simulink model "radial_magnetic_bearing_revised"  (R2021a)
settings: Solver=VariableStepAuto  StartTime=0.0  StopTime=10  RelTol=1e-3
values from neighbouring files (symbols this model uses):
  Ar = [zeros(4) eye(4); zeros(4) -G/M]    [radial_amb.m]
  Br = [zeros(4);B/M]    [radial_amb.m]
  Cr = [C zeros(4)]    [radial_amb.m]
  Dr = zeros(4)    [radial_amb.m]
  Ki = eye(4)*ki    [radial_amb.m]
  KLQR = Nbar    [radial_amb.m]
  Kss = (B*Ks*B')'    [radial_amb.m]
  P0ramb = diag(100*ones(1,8))    [radial_amb.m]
  Qramb = diag(10^-14*ones(1,8))    [radial_amb.m]
  Rramb = diag(10^-14*ones(1,4))    [radial_amb.m]
  sys_dr = c2d(Hsi,dT,'zoh')    [radial_amb.m]
  Tr = inv(T)    [radial_amb.m]
  x0ramb = [0;0;0;0;0;0;0;0]    [radial_amb.m]
libraries: simulink x32
settings Model: Creator=macbookpro  LastModifiedBy=macbookpro

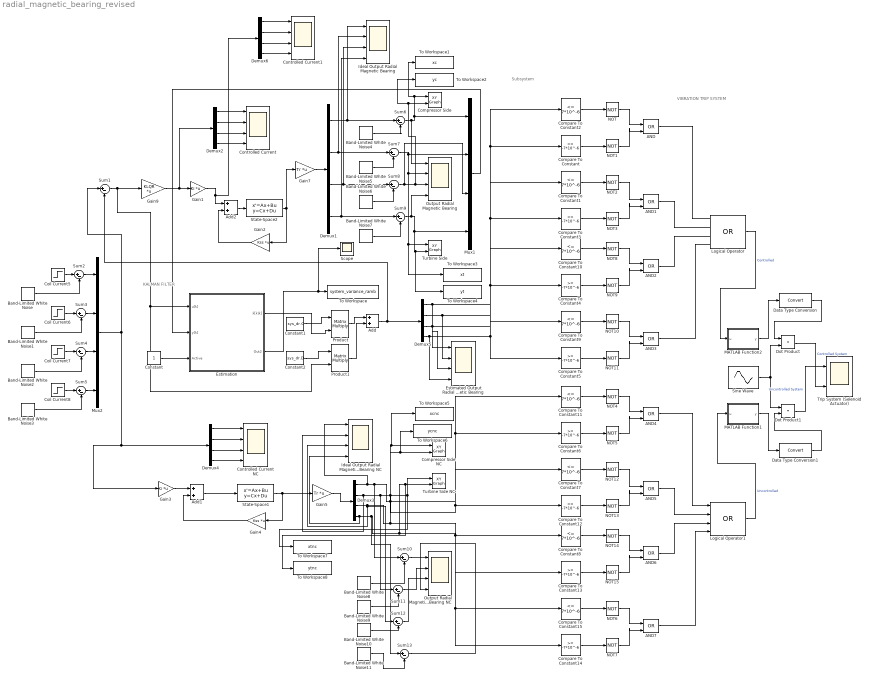
== system radial_magnetic_bearing_revised ==
  note: Subsystem
  note: KALMAN FILTER
  note: VIBRATION TRIP SYSTEM
  AND{,1..7} (8 alike) : Logic  Operator=OR  IconShape=distinctive  AllPortsSameDT=off  OutDataTypeStr=boolean
  Add : Sum
  Add1 : Sum
  Add2 : Sum
  Band-Limited White Noise{,1..3} (4 alike) : simulink/Sources/Band-Limited White Noise  Cov=[0.01]  Ts=0.1  seed=[23341]
  Band-Limited White Noise{4..11} (8 alike) : simulink/Sources/Band-Limited White Noise  Cov=[10^-14]  Ts=0.1  seed=[23341]
  Coil Current{5..8} (4 alike) : Step  After=0.5  SampleTime=0
  Compare To Constant{,3..6,12..14} (8 alike) : simulink/Logic and Bit Operations/Compare To Constant  relop=>=  const=-7*10^-6  OutDataTypeStr=boolean
  Compare To Constant{1..2,7..11,15} (8 alike) : simulink/Logic and Bit Operations/Compare To Constant  relop=<=  const=7*10^-6  OutDataTypeStr=boolean
  "Compressor Side " : simulink/Sinks/XY Graph  xmin=10*-10^-6  xmax=10*10^-6  ymin=10*-10^-6  ymax=10*10^-6  st=0.1
  Compressor Side NC : simulink/Sinks/XY Graph  xmin=10*-10^-6  xmax=10*10^-6  ymin=10*-10^-6  ymax=10*10^-6  st=0.1
  Constant : Constant
  Constant1 : Constant  Value=sys_dr.C  VectorParams1D=off
  Constant2 : Constant  Value=sys_dr.D  VectorParams1D=off
  Controlled Current : Scope  NumInputPorts=4
  Controlled Current NC : Scope  NumInputPorts=4
  Controlled Current1 : Scope  NumInputPorts=4
  Data Type Conversion : DataTypeConversion
  Data Type Conversion1 : DataTypeConversion
  Demux{1..6} (6 alike) : Demux
  Dot Product : DotProduct  InputSameDT=on  OutDataTypeStr=Inherit: Inherit via internal rule
  Dot Product1 : DotProduct  InputSameDT=on  OutDataTypeStr=Inherit: Inherit via internal rule
  Estimated Output Radial Magnetic Bearing : Scope  NumInputPorts=4
  Estimation : Subsystem
  Gain1 : Gain  Gain=Ki  Multiplication=Matrix(K*u)
  Gain2 : Gain  Gain=Kss  Multiplication=Matrix(K*u)
  Gain3 : Gain  Gain=Ki  Multiplication=Matrix(K*u)
  Gain4 : Gain  Gain=Kss  Multiplication=Matrix(K*u)
  Gain5 : Gain  Gain=Tr  Multiplication=Matrix(K*u)
  Gain7 : Gain  Gain=Tr  Multiplication=Matrix(K*u)
  Gain9 : Gain  Gain=KLQR  Multiplication=Matrix(K*u)
  Ideal Output Radial Magnetic Bearing : Scope  NumInputPorts=4
  Ideal Output Radial Magnetic Bearing NC : Scope  NumInputPorts=4
  Logical Operator : Logic  Operator=OR  Inputs=4  IconShape=distinctive  AllPortsSameDT=off  OutDataTypeStr=boolean
  Logical Operator1 : Logic  Operator=OR  Inputs=4  IconShape=distinctive  AllPortsSameDT=off  OutDataTypeStr=boolean
  MATLAB Function1 : MATLAB Function  TreatAsAtomicUnit=on
  MATLAB Function2 : MATLAB Function  TreatAsAtomicUnit=on
  Mux1 : Mux
  Mux2 : Mux
  NOT{,1..15} (16 alike) : Logic  Operator=NOT  IconShape=distinctive  AllPortsSameDT=off  OutDataTypeStr=boolean
  Output Radial Magnetic Bearing : Scope  NumInputPorts=4
  Output Radial Magnetic Bearing NC : Scope  NumInputPorts=4
  Product : Product  Multiplication=Matrix(*)
  Product1 : Product  Multiplication=Matrix(*)
  Scope : Scope
  Sine Wave : Sin  Amplitude=220  Frequency=60  SampleTime=0
  State-Space1 : StateSpace  A=Ar  B=Br  C=Cr  D=Dr  InitialCondition=0
  State-Space2 : StateSpace  A=Ar  B=Br  C=Cr  D=Dr  InitialCondition=10^-7*[1.5 1.5 1.5 1.5 1.5 1.5 1.5 1.5]  ContinuousStateAttributes='posisition'
  Sum{1..13} (13 alike) : Sum  Inputs=|+-
  To Workspace : ToWorkspace  VariableName=system_variance_ramb  SampleTime=-1
      settings: MaxDataPoints=1
  To Workspace1 : ToWorkspace  VariableName=xc  SaveFormat=Timeseries  SampleTime=-1
  To Workspace2 : ToWorkspace  VariableName=yc  SaveFormat=Timeseries  SampleTime=-1
  To Workspace3 : ToWorkspace  VariableName=xt  SaveFormat=Timeseries  SampleTime=-1
  To Workspace4 : ToWorkspace  VariableName=yt  SaveFormat=Timeseries  SampleTime=-1
  To Workspace5 : ToWorkspace  VariableName=xcnc  SaveFormat=Timeseries  SampleTime=-1
  To Workspace6 : ToWorkspace  VariableName=ycnc  SaveFormat=Timeseries  SampleTime=-1
  To Workspace7 : ToWorkspace  VariableName=xtnc  SaveFormat=Timeseries  SampleTime=-1
  To Workspace8 : ToWorkspace  VariableName=ytnc  SaveFormat=Timeseries  SampleTime=-1
  Trip System (Selenoid Actuator) : Scope  NumInputPorts=2
  Turbine Side : simulink/Sinks/XY Graph  xmin=10*-10^-6  xmax=10*10^-6  ymin=10*-10^-6  ymax=10*10^-6  st=0.1
  Turbine Side NC : simulink/Sinks/XY Graph  xmin=10*-10^-6  xmax=10*10^-6  ymin=10*-10^-6  ymax=10*10^-6  st=0.1
  wires:
  State-Space2/1 -> Gain7/1, Gain2/1
  Gain2/1 -> Add2/2
  Add2/1 -> State-Space2/1
  Demux2/1 -> Controlled Current/1
  Demux2/2 -> Controlled Current/2
  Demux2/3 -> Controlled Current/3
  Demux2/4 -> Controlled Current/4
  Coil Current5/1 -> Sum2/1
  Coil Current8/1 -> Sum5/1
  Coil Current7/1 -> Sum4/1
  Coil Current6/1 -> Sum3/1
  Sum2/1 -> Mux2/1
  Sum3/1 -> Mux2/2
  Sum4/1 -> Mux2/3
  Sum5/1 -> Mux2/4
  Band-Limited White Noise/1 -> Sum2/2
  Band-Limited White Noise3/1 -> Sum5/2
  Band-Limited White Noise2/1 -> Sum4/2
  Band-Limited White Noise1/1 -> Sum3/2
  Add1/1 -> State-Space1/1
  Demux4/4 -> Controlled Current NC/4
  Gain4/1 -> Add1/2
  Demux4/2 -> Controlled Current NC/2
  State-Space1/1 -> Gain4/1, Gain5/1
  Gain5/1 -> Demux3/1
  Gain3/1 -> Add1/1
  Mux2/1 -> Gain3/1, Demux4/1, Sum1/1
  Demux4/3 -> Controlled Current NC/3
  Demux4/1 -> Controlled Current NC/1
  Demux1/1 -> Ideal Output Radial Magnetic Bearing/1, Sum6/1
  Band-Limited White Noise5/1 -> Sum7/2
  Demux1/3 -> Ideal Output Radial Magnetic Bearing/3, Sum8/1
  Demux1/2 -> Ideal Output Radial Magnetic Bearing/2, Sum7/1
  Band-Limited White Noise7/1 -> Sum9/2
  Band-Limited White Noise6/1 -> Sum8/2
  Demux1/4 -> Ideal Output Radial Magnetic Bearing/4, Sum9/1
  Band-Limited White Noise4/1 -> Sum6/2
  Sum6/1 -> "Compressor Side "/1, To Workspace1/1, Mux1/1, Output Radial Magnetic Bearing/1
  Sum7/1 -> To Workspace3/1, Turbine Side/1, Output Radial Magnetic Bearing/2, Mux1/2
  Sum8/1 -> "Compressor Side "/2, To Workspace2/1, Output Radial Magnetic Bearing/3, Mux1/3
  Sum9/1 -> To Workspace4/1, Turbine Side/2, Mux1/4, Output Radial Magnetic Bearing/4
  Sum1/1 -> Product1/2, Estimation/1(u[k]), Gain9/1
  Mux1/1 -> Estimation/2(y[k])
  Product1/1 -> Add/2
  Product/1 -> Add/1
  Estimation/1(x̂[k|k]) -> Product/2
  Estimation/2(Out2) -> Scope/1, To Workspace/1
  Add/1 -> Demux5/1, Sum1/2
  Constant/1 -> Estimation/3(Active)
  Constant1/1 -> Product/1
  Constant2/1 -> Product1/1
  Gain7/1 -> Demux1/1
  Gain9/1 -> Gain1/1, Demux2/1
  AND5/1 -> Logical Operator1/2
  Data Type Conversion/1 -> Dot Product/1
  AND1/1 -> Logical Operator/2
  Compare To Constant10/1 -> NOT8/1
  Compare To Constant14/1 -> NOT7/1
  Logical Operator/1 -> MATLAB Function2/1(u)  "Controlled"
  NOT11/1 -> AND3/2
  AND3/1 -> Logical Operator/4
  AND4/1 -> Logical Operator1/1
  Demux5/3 -> Compare To Constant4/1, Compare To Constant10/1, Estimated Output Radial Magnetic Bearing/3
  NOT2/1 -> AND1/1
  Demux5/1 -> Compare To Constant/1, Compare To Constant2/1, Estimated Output Radial Magnetic Bearing/1
  Sine Wave/1 -> Dot Product1/1, Dot Product/2
  AND7/1 -> Logical Operator1/4
  Compare To Constant/1 -> NOT1/1
  Logical Operator1/1 -> MATLAB Function1/1(u)  "Uncontrolled"
  NOT9/1 -> AND2/2
  NOT4/1 -> AND4/1
  NOT10/1 -> AND3/1
  Compare To Constant5/1 -> NOT11/1
  NOT14/1 -> AND6/1
  Compare To Constant1/1 -> NOT2/1
  NOT6/1 -> AND7/1
  NOT8/1 -> AND2/1
  Compare To Constant2/1 -> NOT/1
  Compare To Constant11/1 -> NOT4/1
  Demux5/4 -> Compare To Constant9/1, Compare To Constant5/1, Estimated Output Radial Magnetic Bearing/4
  Compare To Constant7/1 -> NOT12/1
  NOT3/1 -> AND1/2
  NOT1/1 -> AND/2
  AND/1 -> Logical Operator/1
  NOT13/1 -> AND5/2
  Compare To Constant15/1 -> NOT6/1
  Compare To Constant9/1 -> NOT10/1
  NOT12/1 -> AND5/1
  Compare To Constant6/1 -> NOT5/1
  AND2/1 -> Logical Operator/3
  MATLAB Function2/1(y) -> Data Type Conversion/1
  Compare To Constant3/1 -> NOT3/1
  Compare To Constant12/1 -> NOT13/1
  NOT15/1 -> AND6/2
  NOT5/1 -> AND4/2
  Demux5/2 -> Compare To Constant3/1, Compare To Constant1/1, Estimated Output Radial Magnetic Bearing/2
  Compare To Constant4/1 -> NOT9/1
  Dot Product/1 -> Trip System (Selenoid Actuator)/2  "Controlled System"
  AND6/1 -> Logical Operator1/3
  Compare To Constant13/1 -> NOT15/1
  Data Type Conversion1/1 -> Dot Product1/2
  MATLAB Function1/1(y) -> Data Type Conversion1/1
  Dot Product1/1 -> Trip System (Selenoid Actuator)/1  "Uncontrolled System"
  NOT/1 -> AND/1
  NOT7/1 -> AND7/2
  Compare To Constant8/1 -> NOT14/1
  Demux3/4 -> Sum13/1, Compare To Constant14/1, Compare To Constant15/1, To Workspace8/1, Turbine Side NC/2, Ideal Output Radial Magnetic Bearing NC/4
  Band-Limited White Noise8/1 -> Sum10/2
  Demux3/3 -> Sum12/1, Ideal Output Radial Magnetic Bearing NC/3, Compare To Constant13/1, Compare To Constant8/1, To Workspace6/1, Compressor Side NC/2
  Band-Limited White Noise11/1 -> Sum13/2
  Band-Limited White Noise10/1 -> Sum12/2
  Band-Limited White Noise9/1 -> Sum11/2
  Demux3/2 -> Ideal Output Radial Magnetic Bearing NC/2, Sum11/1, Compare To Constant12/1, Compare To Constant7/1, Turbine Side NC/1, To Workspace7/1
  Demux3/1 -> Ideal Output Radial Magnetic Bearing NC/1, Sum10/1, Compare To Constant6/1, Compare To Constant11/1, To Workspace5/1, Compressor Side NC/1
  Sum10/1 -> Output Radial Magnetic Bearing NC/1
  Sum11/1 -> Output Radial Magnetic Bearing NC/2
  Sum12/1 -> Output Radial Magnetic Bearing NC/3
  Sum13/1 -> Output Radial Magnetic Bearing NC/4
  Demux6/3 -> Controlled Current1/3
  Demux6/2 -> Controlled Current1/2
  Gain1/1 -> Demux6/1, Add2/1
  Demux6/1 -> Controlled Current1/1
  Demux6/4 -> Controlled Current1/4

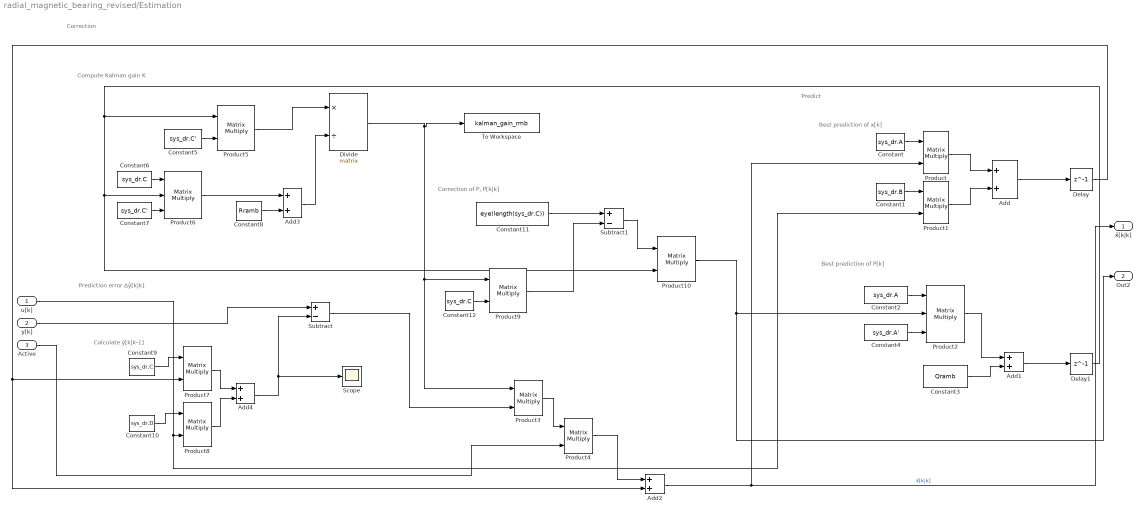
== system radial_magnetic_bearing_revised/Estimation ==
  note: Best prediction of x[k]
  note: Predict
  note: Best prediction of P[k]
  note: Correction of P, P[k|k]
  note: Prediction error Δŷ[k|k]
  note: Compute Kalman gain K
  note: Correction
  note: Calculate ŷ[k|k-1]
  u[k] : Inport
  y[k] : Inport  Port=2
  Active : Inport  Port=3
  Add{,1..4} (5 alike) : Sum
  Constant : Constant  Value=sys_dr.A  VectorParams1D=off
  Constant1 : Constant  Value=sys_dr.B  VectorParams1D=off
  Constant10 : Constant  Value=sys_dr.D  VectorParams1D=off
  Constant11 : Constant  Value=eye(length(sys_dr.C))  VectorParams1D=off
  Constant12 : Constant  Value=sys_dr.C  VectorParams1D=off
  Constant2 : Constant  Value=sys_dr.A  VectorParams1D=off
  Constant3 : Constant  Value=Qramb  VectorParams1D=off
  Constant4 : Constant  Value=sys_dr.A'  VectorParams1D=off
  Constant5 : Constant  Value=sys_dr.C'  VectorParams1D=off
  Constant6 : Constant  Value=sys_dr.C  VectorParams1D=off
  Constant7 : Constant  Value=sys_dr.C'  VectorParams1D=off
  Constant8 : Constant  Value=Rramb  VectorParams1D=off
  Constant9 : Constant  Value=sys_dr.C  VectorParams1D=off
  Delay : Delay  DelayLength=1  InitialCondition=x0ramb
  Delay1 : Delay  DelayLength=1  InitialCondition=P0ramb
  Divide : Product  Inputs=*/  Multiplication=Matrix(*)
  Product{,1,3..5,7..10} (9 alike) : Product  Multiplication=Matrix(*)
  Product2 : Product  Inputs=3  Multiplication=Matrix(*)
  Product6 : Product  Inputs=3  Multiplication=Matrix(*)
  Scope : Scope
  Subtract : Sum  Inputs=+-
  Subtract1 : Sum  Inputs=+-
  To Workspace : ToWorkspace  VariableName=kalman_gain_rmb  SampleTime=-1
      settings: MaxDataPoints=1
  x̂[k|k] : Outport
  Out2 : Outport  Port=2
  wires:
  Constant4/1 -> Product2/3
  Constant/1 -> Product/1
  Product1/1 -> Add/2
  Constant11/1 -> Subtract1/1
  Constant6/1 -> Product6/1
  Constant12/1 -> Product9/2
  Constant2/1 -> Product2/1
  Constant3/1 -> Add1/2
  Product9/1 -> Subtract1/2
  Constant9/1 -> Product7/1
  Constant8/1 -> Add3/2
  Add3/1 -> Divide/2
  Product3/1 -> Product4/1
  u[k]/1 -> Product8/2, Product1/2
  Add/1 -> Delay/1
  Product8/1 -> Add4/2
  Add4/1 -> Subtract/2, Scope/1
  Constant5/1 -> Product5/2
  Delay/1 -> Add2/2, Product7/2
  Add2/1 -> Product/2, x̂[k|k]/1  "x̂[k|k]"
  Constant1/1 -> Product1/1
  Product/1 -> Add/1
  Active/1 -> Product4/2
  Subtract/1 -> Product3/2
  Add1/1 -> Delay1/1
  Product2/1 -> Add1/1
  Constant7/1 -> Product6/3
  Product4/1 -> Add2/1
  Delay1/1 -> Product6/2, Product10/2, Product5/1
  Product6/1 -> Add3/1
  Divide/1 -> To Workspace/1, Product3/1, Product9/1
  y[k]/1 -> Subtract/1
  Product5/1 -> Divide/1
  Constant10/1 -> Product8/1
  Product7/1 -> Add4/1
  Product10/1 -> Out2/1, Product2/2
  Subtract1/1 -> Product10/1

== matlab function radial_magnetic_bearing_revised/MATLAB Function2 ==
  data: u input; y output
%MEALY FINITE STATE MACHINE
function y = TRIP(u)
if(u==0)
    u=false;
else
    u=true
end

S1=0;
S2=1;
persistent state;
if isempty(state)
    state=S1;
end

switch(state)
    case S1,
        if(u==false)
            y=false;
            state=S1;
        else
            y=true;
            state=S2;
        end
        
    case S2,
        if(u==false)
            y=true;
            state=S2;
        else
            y=false;
            state=S2;
        end
end
if state==S1
    y=false
else
    state==S2
    y=true
end
end

== matlab function radial_magnetic_bearing_revised/MATLAB Function1 ==
  data: u input; y output
function y = TRIP(u)
if(u==0)
    u=false;
else
    u=true
end

S1=0;
S2=1;
persistent state;
if isempty(state)
    state=S1;
end

switch(state)
    case S1,
        if(u==false)
            y=false;
            state=S1;
        else
            y=true;
            state=S2;
        end
        
    case S2,
        if(u==false)
            y=true;
            state=S2;
        else
            y=false;
            state=S2;
        end
end
if state==S1
    y=false
else
    state==S2
    y=true
end
end
